simulink model "PFC_FutureSetpoint"  (R2015a)
settings: Solver=ode45  StartTime=0.0  StopTime=20  RelTol=1e-3
values from neighbouring files (symbols this model uses):
  Ad = sysd.a    [PFC_config.m]
  Bd = sysd.b    [PFC_config.m]
  Cd = sysd.c    [PFC_config.m]
  Dd = sysd.d    [PFC_config.m]
  dSamplingPeriod = 0.1    [PFC_config.m]
  SF = zeros( 3, 3 )    [PFC_config.m]
  SWITCH = 0    [PFC_config.m]
  sys = tf( [ 1 ], [ 1, 2*0.5, 1 ] )    [PFC_config.m]
  TCLRT = 1.0    (= 1)    [PFC_config.m]
settings Model: Creator=hamada  LastModifiedBy=hamada

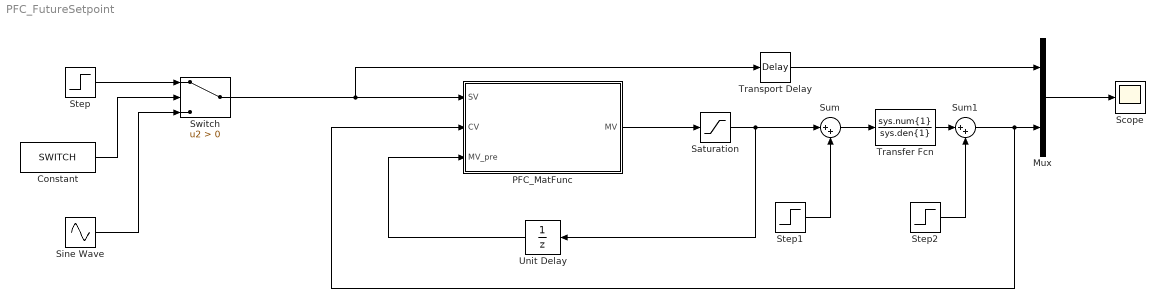
== system PFC_FutureSetpoint ==
  Constant : Constant  Value=SWITCH
  Mux : Mux  Inputs=2
  PFC_MatFunc : MATLAB Function  TreatAsAtomicUnit=on
  Saturation : Saturate  UpperLimit=3  LowerLimit=-3
  Scope : Scope
      settings: SaveName=PFC_Output
  Sine Wave : Sin  SampleTime=0
  Step : Step  SampleTime=0
  Step1 : Step  Time=14  After=0.3  SampleTime=0
  Step2 : Step  Time=8  After=0.3  SampleTime=0
  Sum : Sum  Inputs=|++
  Sum1 : Sum  Inputs=|++
  Switch : Switch  Criteria=u2 > Threshold
  Transfer Fcn : TransferFcn  Numerator=sys.num{1}  Denominator=sys.den{1}
  Transport Delay : TransportDelay  DelayTime=h(end)*dSamplingPeriod
  Unit Delay : UnitDelay  SampleTime=dSamplingPeriod
  wires:
  Unit Delay/1 -> PFC_MatFunc/3(MV_pre)
  PFC_MatFunc/1(MV) -> Saturation/1
  Saturation/1 -> Sum/1, Unit Delay/1
  Switch/1 -> Transport Delay/1, PFC_MatFunc/1(SV)
  Sum1/1 -> Mux/2, PFC_MatFunc/2(CV)
  Mux/1 -> Scope/1
  Step/1 -> Switch/1
  Sine Wave/1 -> Switch/3
  Constant/1 -> Switch/2
  Transport Delay/1 -> Mux/1
  Sum/1 -> Transfer Fcn/1
  Step1/1 -> Sum/2
  Transfer Fcn/1 -> Sum1/1
  Step2/1 -> Sum1/2

== matlab function PFC_FutureSetpoint/PFC_MatFunc ==
  settings: updateMethod=DISCRETE  sampleTime=dSamplingPeriod
  data: SV input double; MV output double; CV input double; MV_pre input double; Ad parameter double; Bd parameter double; Cd parameter double; Dd parameter double; SF parameter double; TCLRT parameter double; dSamplingPeriod parameter double
function MV = PFC_MatFunc( SV, CV, MV_pre, Ad, Bd, Cd, Dd, SF, TCLRT, dSamplingPeriod )
    %#codegen
    persistent xm;
    persistent SV_buff;
    
    if ( isempty( xm ) )
        xm = zeros( length( Ad(1,:) ), 1 );
    end

    if ( isempty( SV_buff ) )
        SV_buff = zeros( ( ceil( TCLRT / ( dSamplingPeriod ) ) + 1 ), 1 );
    end

    % 将来の目標値を利用して位相補償
    for cnt = 1:( length( SV_buff ) - 1 )
        SV_buff(cnt) = SV_buff(cnt+1);
    end
    SV_buff(end) = SV;

    xm = Ad * xm + Bd * MV_pre;
    ym = Cd * xm + Dd * MV_pre;
   
   
    h1 = ceil( TCLRT / ( dSamplingPeriod * 3 ) );
    h2 = ceil( TCLRT / ( dSamplingPeriod * 2 ) );
    h3 = ceil( TCLRT / ( dSamplingPeriod * 1 ) );

    SL = [
        Cd * Ad^h1 * xm;
        Cd * Ad^h2 * xm;
        Cd * Ad^h3 * xm;
    ];
   
    lh = [ ...
        ( 1 - exp( -3 * h1 * dSamplingPeriod / TCLRT ) );
        ( 1 - exp( -3 * h2 * dSamplingPeriod / TCLRT ) );
        ( 1 - exp( -3 * h3 * dSamplingPeriod / TCLRT ) );
    ];
   
    SV_future = [
        SV_buff(h1+1) - SV_buff(1);
        SV_buff(h2+1) - SV_buff(1);
        SV_buff(h3+1) - SV_buff(1);
    ];

    buff  = SF \ ( SV_future + ( SV_buff(1) - CV ) .* lh - SL + ym );
    MV = buff(1);
end
